simulink model "Lab1_Starter"  (R2014a)
settings: Solver=ode45  StartTime=0.0  StopTime=10.0  RelTol=1e-3
settings Model: Creator=Rebecca  LastModifiedBy=Rebecca

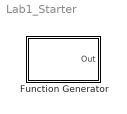
== system Lab1_Starter ==
  Function Generator : Subsystem  TreatAsAtomicUnit=on  mask{funcType=Triangle Wave, mag=1, freq=.5}
      mask prompts: funcType "Function Type"; mag "Peak-to-Peak Amplitude (Volts)"; freq "Frequency (Hertz)"
      mask help: Generates either a square wave or a triangle wave based on the selections below.
      mask TypeOptions funcType: Triangle Wave | Square Wave

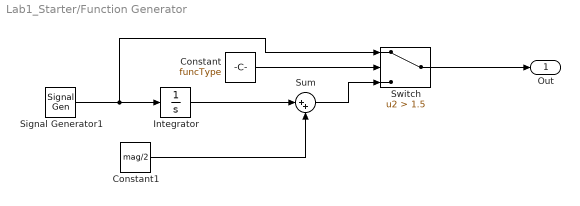
== system Lab1_Starter/Function Generator ==
  Constant : Constant  Value=funcType
  Constant1 : Constant  Value=mag/2
  Integrator : Integrator
  Signal Generator1 : SignalGenerator  WaveForm=square  Amplitude=mag  Frequency=freq
  Sum : Sum  Inputs=|++
  Switch : Switch  Criteria=u2 > Threshold  Threshold=1.5
  Out : Outport
  wires:
  Switch/1 -> Out/1
  Signal Generator1/1 -> Switch/1, Integrator/1
  Constant/1 -> Switch/2
  Integrator/1 -> Sum/1
  Sum/1 -> Switch/3
  Constant1/1 -> Sum/2
